simulink model "sgMdl_IO3xx_Serial_Loopback_Halfduplex"  (R2024b)
settings: Solver=FixedStepAuto  StartTime=0.0  StopTime=inf  RelTol=1e-3  EnableMultiTasking=on
undefined symbols (not defined in the file): Pull, pull, up
libraries: speedgoatlib_fpga_serial x6, simulink x2, speedgoatlib_interrupt x1, speedgoatlib_fpga x1
Description:
  | IO3xx Serial - Loopback Halfduplex
settings Model: ModifiedByFormat=Speedgoat  SimulationMode=external  ExtModeTrigDuration=100000  Creator=Speedgoat  LastModifiedBy=Speedgoat
settings SolverCC: ConcurrentTasks=on  AlgebraicLoopSolver=TrustRegion  PositivePriorityOrder=on  InsertRTBMode=Never (minimum delay)
settings DataIOCC: SaveFormat=Array  SaveState=on  SignalLoggingName=logsOut
settings OptimizationCC: BlockReduction=off  BooleanDataType=off  OptimizeBlockIOStorage=off  BufferReuse=off  ReuseModelBlockBuffer=off  GlobalBufferReuse=off  ExpressionFolding=off  LocalBlockOutputs=off  InitFltsAndDblsToZero=on  OptimizeDataStoreBuffers=off  BusAssignmentInplaceUpdate=off
settings DebuggingCC: SaveWithParameterizedLinksMsg=none  UnderspecifiedInitializationDetection=Classic  MergeDetectMultiDrivingBlocksExec=none  CheckExecutionContextPreStartOutputMsg=on  SignalResolutionControl=TryResolveAllWithWarning  TasksWithSamePriorityMsg=none  UnconnectedInputMsg=warning  UnconnectedOutputMsg=warning  UnconnectedLineMsg=warning  SFUnexpectedBacktrackingDiag=warning  SFNoUnconditionalDefaultTransitionDiag=warning  SFExecutionAtInitializationDiag=none  ArithmeticOperatorsInVariantConditions=warning
settings HardwareCC: ProdBitPerLong=64  ProdLongLongMode=on  ProdHWDeviceType=Intel->x86-64 (Linux 64)
settings ModelReferenceCC: EnableRefExpFcnMdlSchedulingChecks=on  PropagateSignalLabelsOutOfModel=off
settings SFSimCC: SimUseLocalCustomCode=off  SimTargetLang=C++
settings RTWCC: Description=Speedgoat Real-Time Target Machine  SystemTargetFile=speedgoat.tlc  TemplateMakefile=slrealtime_default_tmf  PostCodeGenCommand=sg.model.build.makeCfg(bdroot, buildInfo);  RTWUseLocalCustomCode=off  Toolchain=Simulink Real-Time Toolchain  BuildConfiguration=Faster Runs  TargetLang=C++  GPUComputeCapability=3.5  DLArmComputeVersion=19.05
settings CodeAppCC: StateflowObjectComments=on
settings SimulinkRealTimeTargetCC: SubcomponentCodeInterfacePackaging=Reusable function  MATLABClassNameForMDSCustomization=Simulink.SoftwareTarget.GRTCustomization  InstructionSetFMA=off  LogToMDFFile=off  SLRTFileLogMaxRuns=10  UseGCCFastMath=on
settings ConfigComp: CovMetricSettings=dw  CovSaveCumulativeToWorkspaceVar=on  CovSaveSingleToWorkspaceVar=on  CovExternalEMLEnable=off  CovSFcnEnable=off  CovBoundaryAbsTol=1.0e-5

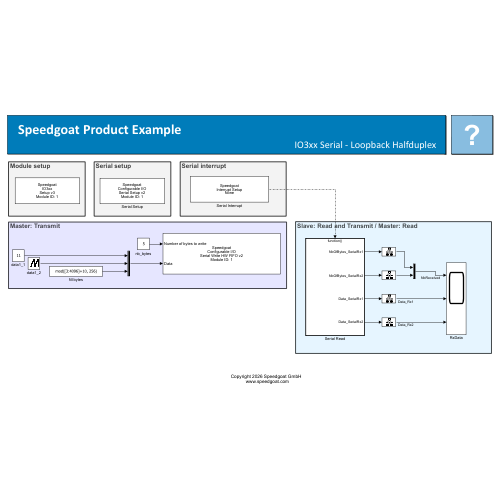
[thumbnail: Simulink's stored preview of the top-level diagram]
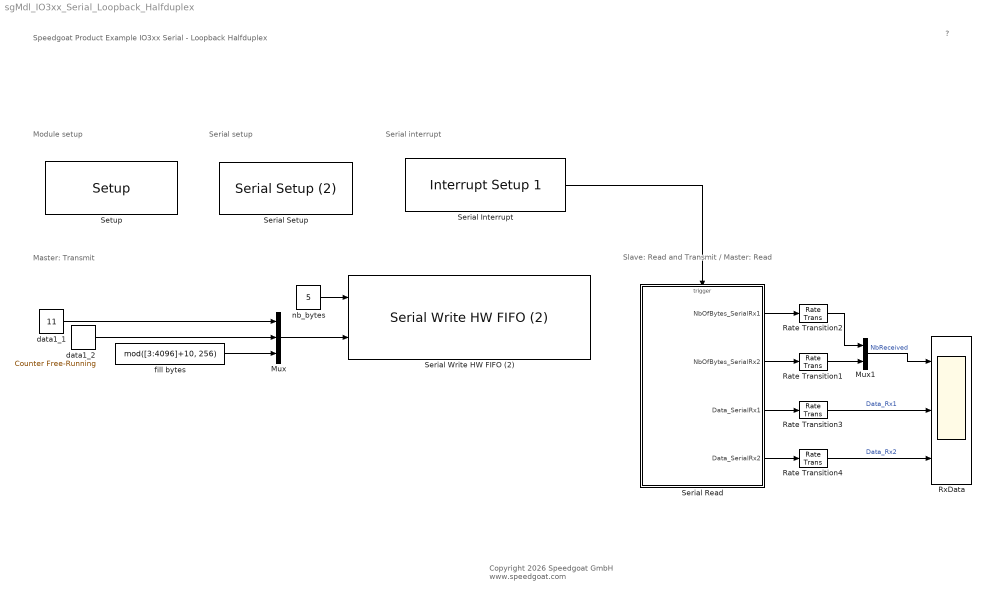
== system sgMdl_IO3xx_Serial_Loopback_Halfduplex ==
  note: Slave: Read and Transmit / Master: Read
  note: Master: Transmit
  note: Module setup
  note: Serial setup
  note: Serial interrupt
  note: Speedgoat Product Example
      | IO3xx Serial - Loopback Halfduplex
  note: ?
  note: Copyright 2026 Speedgoat GmbH
      |  www.speedgoat.com
  Mux : Mux  Inputs=3
  Mux1 : Mux  Inputs=2
  Rate Transition{1..4} (4 alike) : RateTransition  Deterministic=off
  RxData : Scope  NumInputPorts=3
  Serial Interrupt : speedgoatlib_interrupt/Interrupt Setup 1  parModuleTrigger=off  parPollingMode=off  parPriorityConf=High  parPriority=254  confStartFcn=IO324_200k_SERIAL_start_public  confStopFcn=IO324_200k_SERIAL_stop_public  confIsrFcn=IO324_200k_SERIAL_isr_public  confMapFcn=IO324_200k_SERIAL_map_public  confHookFile=io324_200k_serial_int_hooks.c  confIrqNr=-1  confIsPolling=off  confModID=16776961  confSelectedInt=None  confSelectedId=[]  confSelectedChannel=[]  confData=[]  confForcePollingMode=off
  Serial Read : Subsystem  TreatAsAtomicUnit=on
  Serial Setup : speedgoatlib_fpga_serial/Serial Setup (2)  id=1  channel=[1, 2]  bitrate=[1e6]  bitrate_effective=[996.3243e3, 996.3243e3]  bitrate_error=[-0.36757, -0.36757]  parity_mode=No parity  data_length=[8]  stop_length=[2]  enable_half_duplex=[0]  rx_character_timeout=[1 1]
      settings: SourceProductName=Simulink Real-Time: Speedgoat I/O Blockset
  Serial Write HW FIFO (2) : speedgoatlib_fpga_serial/Serial Write HW FIFO (2)  id=1  channel=1  ts=-1  data_length=8
      settings: SourceProductName=Simulink Real-Time: Speedgoat I/O Blockset
  Setup : speedgoatlib_fpga/Setup/Setup  board=Please select...  id=1  pciSlot=-1  device_id=1  bitstreamFilePath=C:\Work\SVN\Speedgoatlib\releases\10.0.0\product_examples\IO3xx_Serial  bitstreamFile=Please select...  fpgaFreq=[73728000 100000000]  enableDma=off  rearEnb_1=off  rearIO_1=None  rearEnb_2=off  rearIO_2=None  ProgSpiFlash=off  ProgBPIFlash=off  useFpgaDmaController=off  dmaTrigDropdown=Model Step  dmaTrigSelect=0  dmaStopOnOverload=on  dmaModeSequential=on  dmaModeParallel=off  PullRPort15=pull-up 3.3V  PullRPort31=pull-up 3.3V  PullRPort47=pull-up 3.3V  PullRPort63=pull-up 3.3V  diffLineTermination_1=on  diffLineTermination_2=on  diffLineTermination_3=on  diffLineTermination_4=on  diffLineTermination_5=on  diffLineTermination_6=on  diffLineTermination_7=on  diffLineTermination_8=on  diffLineTermination_9=on  diffLineTermination_10=on  diffLineTermination_11=on  diffLineTermination_12=on  diffLineTermination_13=on  diffLineTermination_14=on  diffLineTermination_15=on  diffLineTermination_16=on  diffLineTermination_17=on  diffLineTermination_18=on  diffLineTermination_19=on  diffLineTermination_20=on  diffLineTermination_21=on  diffLineTermination_22=on  diffLineTermination_23=on  diffLineTermination_24=on  diffLineTermination_25=on  diffLineTermination_26=on  diffLineTermination_27=on  diffLineTermination_28=on  diffLineTermination_29=on  diffLineTermination_30=on  diffLineTermination_31=on  diffLineTermination_32=on  ioVoltageDropDown1=3.3V  pullResistorDropDown1_1=Pull-up  pullResistorDropDown1_2=Pull-up  pullResistorDropDown1_3=Pull-up  pullResistorDropDown1_4=Pull-up  pullResistorDropDown1_5=Pull-up  pullResistorDropDown1_6=Pull-up  pullResistorDropDown1_7=Pull-up  pullResistorDropDown1_8=Pull-up  ttlIsImplementedCheckBox1=off  pullResistorDropDown2=Pull-up  ioVoltageDropDown2=3.3V  ttlIsImplementedCheckBox2=off  pullResistorDropDown3=Pull-up  ioVoltageDropDown3=3.3V  ttlIsImplementedCheckBox3=off  pullResistorDropDown4=Pull-up  ioVoltageDropDown4=3.3V  ttlIsImplementedCheckBox4=off  pullResistorDropDown5=Pull-up  ioVoltageDropDown5=3.3V  ttlIsImplementedCheckBox5=off  pullResistorDropDown6=Pull-up  ioVoltageDropDown6=3.3V  ttlIsImplementedCheckBox6=off  pullResistorDropDown7=Pull-up  ioVoltageDropDown7=3.3V  ttlIsImplementedCheckBox7=off  pullResistorDropDown8=Pull-up  ioVoltageDropDown8=3.3V  ttlIsImplementedCheckBox8=off  terminationCheckBox1=off  terminationCheckBox2=off  terminationCheckBox3=off  terminationCheckBox4=off  diffIsImplementedCheckBox1=off  terminationCheckBox5=off  terminationCheckBox6=off  terminationCheckBox7=off  terminationCheckBox8=off  diffIsImplementedCheckBox2=off  terminationCheckBox9=off  terminationCheckBox10=off  terminationCheckBox11=off  terminationCheckBox12=off  diffIsImplementedCheckBox3=off  terminationCheckBox13=off  terminationCheckBox14=off  terminationCheckBox15=off  terminationCheckBox16=off  diffIsImplementedCheckBox4=off  terminationCheckBox17=off  terminationCheckBox18=off  terminationCheckBox19=off  terminationCheckBox20=off  diffIsImplementedCheckBox5=off  terminationCheckBox21=off  terminationCheckBox22=off  terminationCheckBox23=off  terminationCheckBox24=off  diffIsImplementedCheckBox6=off  terminationCheckBox25=off  terminationCheckBox26=off  terminationCheckBox27=off  terminationCheckBox28=off  diffIsImplementedCheckBox7=off  terminationCheckBox29=off  terminationCheckBox30=off  terminationCheckBox31=off  terminationCheckBox32=off  diffIsImplementedCheckBox8=off  PullRPort0_1=pull-up  VioPort0_1=3.3V  PullRPort1_1=pull-up  VioPort1_1=3.3V  PullRPort2_1=pull-up  VioPort2_1=3.3V  PullRPort3_1=pull-up  VioPort3_1=3.3V  PullRPort4_1=pull-up  VioPort4_1=3.3V  PullRPort5_1=pull-up  VioPort5_1=3.3V  PullRPort6_1=pull-up  VioPort6_1=3.3V  diffLineTermination_rear1_1=on  diffLineTermination_rear1_2=on  diffLineTermination_rear1_3=on  diffLineTermination_rear1_4=on  diffLineTermination_rear1_5=on  diffLineTermination_rear1_6=on  diffLineTermination_rear1_7=on  diffLineTermination_rear1_8=on  PullRPort0_2=pull-up  VioPort0_2=3.3V  PullRPort1_2=pull-up  VioPort1_2=3.3V  PullRPort2_2=pull-up  VioPort2_2=3.3V  PullRPort3_2=pull-up  VioPort3_2=3.3V  PullRPort4_2=pull-up  VioPort4_2=3.3V  PullRPort5_2=pull-up  VioPort5_2=3.3V  PullRPort6_2=pull-up  VioPort6_2=3.3V  diffLineTermination_rear2_1=on  diffLineTermination_rear2_2=on  diffLineTermination_rear2_3=on  diffLineTermination_rear2_4=on  diffLineTermination_rear2_5=on  diffLineTermination_rear2_6=on  diffLineTermination_rear2_7=on  diffLineTermination_rear2_8=on
      settings: SourceProductName=Simulink Real-Time: Speedgoat I/O Blockset
  data1_1 : Constant  Value=11  OutDataTypeStr=Inherit: Inherit via back propagation
  data1_2 : simulink/Sources/Counter Free-Running  NumBits=8  tsamp=1e-3
  fill bytes : Constant  Value=mod([3:4096]+10, 256)  OutDataTypeStr=Inherit: Inherit via back propagation
  nb_bytes : Constant  Value=5  OutDataTypeStr=Inherit: Inherit via back propagation
      mask help: Speedgoat Utility Block<br>Interrupt Setup - Configure Speedgoat I/O Module interrupts<br><br>&copy; 2007 - 2026, Speedgoat GmbH, <a href="matlab: web('www.speedgoat.com','-browser');">www.speedgoat.com</a>
      mask Help: eval('sg.utils.help.show(''io_main/refentry_ref_interrupt_setup'');')
  wires:
  data1_1/1 -> Mux/1
  nb_bytes/1 -> Serial Write HW FIFO (2)/1
  Mux/1 -> Serial Write HW FIFO (2)/2
  Serial Read/4(Data_SerialRx2) -> Rate Transition4/1
  Serial Read/2(NbOfBytes_SerialRx2) -> Rate Transition1/1
  fill bytes/1 -> Mux/3
  Serial Read/1(NbOfBytes_SerialRx1) -> Rate Transition2/1
  Serial Read/3(Data_SerialRx1) -> Rate Transition3/1
  Serial Interrupt/1 -> Serial Read/Trigger
  data1_2/1 -> Mux/2
  Rate Transition4/1 -> RxData/3  "Data_Rx2"
  Rate Transition3/1 -> RxData/2  "Data_Rx1"
  Rate Transition1/1 -> Mux1/2
  Rate Transition2/1 -> Mux1/1
  Mux1/1 -> RxData/1  "NbReceived"

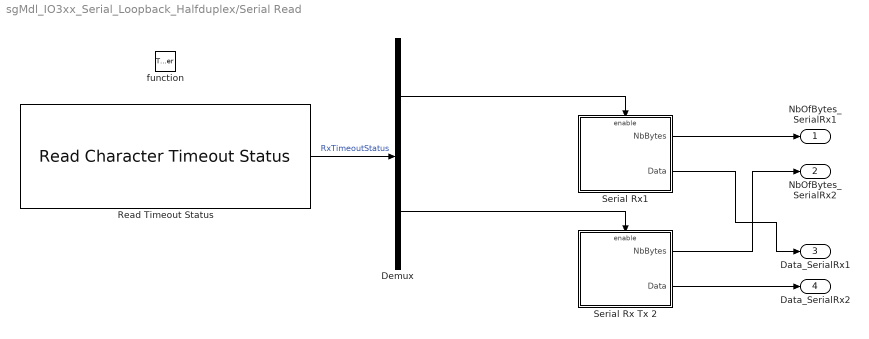
== system sgMdl_IO3xx_Serial_Loopback_Halfduplex/Serial Read ==
  function : TriggerPort  TriggerType=function-call  VariantControl=Variant
  Demux : Demux  Outputs=2
  Read Timeout Status : speedgoatlib_fpga_serial/Read Character Timeout Status  id=1  channel=[1, 2]  ts=-1
      settings: SourceProductName=Simulink Real-Time: Speedgoat I/O Blockset
  Serial Rx Tx 2 : Subsystem  TreatAsAtomicUnit=on
  Serial Rx1 : Subsystem  TreatAsAtomicUnit=on
  NbOfBytes_SerialRx1 : Outport
  NbOfBytes_SerialRx2 : Outport  Port=2
  Data_SerialRx1 : Outport  Port=3
  Data_SerialRx2 : Outport  Port=4
  wires:
  Serial Rx Tx 2/2(Data) -> Data_SerialRx2/1
  Serial Rx Tx 2/1(NbBytes) -> NbOfBytes_SerialRx2/1
  Demux/1 -> Serial Rx1/Enable
  Demux/2 -> Serial Rx Tx 2/Enable
  Read Timeout Status/1 -> Demux/1  "RxTimeoutStatus"
  Serial Rx1/1(NbBytes) -> NbOfBytes_SerialRx1/1
  Serial Rx1/2(Data) -> Data_SerialRx1/1

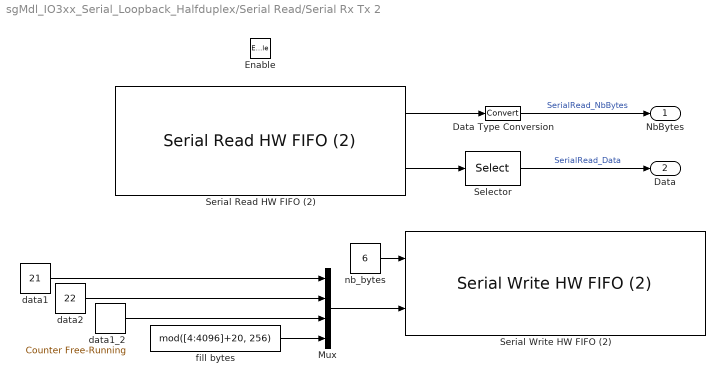
== system sgMdl_IO3xx_Serial_Loopback_Halfduplex/Serial Read/Serial Rx Tx 2 ==
  Enable : EnablePort
  Data Type Conversion : DataTypeConversion  SaturateOnIntegerOverflow=off  RndMeth=Floor
  Mux : Mux
  Selector : Selector  InputPortWidth=4096  IndexOptions=Index vector (dialog)  Indices=[1:5]  OutputSizes=1
  Serial Read HW FIFO (2) : speedgoatlib_fpga_serial/Serial Read HW FIFO (2)  id=1  channel=2  ts=-1  data_length=8
      settings: SourceProductName=Simulink Real-Time: Speedgoat I/O Blockset
  Serial Write HW FIFO (2) : speedgoatlib_fpga_serial/Serial Write HW FIFO (2)  id=1  channel=2  ts=-1  data_length=8
      settings: SourceProductName=Simulink Real-Time: Speedgoat I/O Blockset
  data1 : Constant  Value=21  OutDataTypeStr=Inherit: Inherit via back propagation  SampleTime=-1
  data1_2 : simulink/Sources/Counter Free-Running  NumBits=8  tsamp=-1
  data2 : Constant  Value=22  OutDataTypeStr=Inherit: Inherit via back propagation  SampleTime=-1
  fill bytes : Constant  Value=mod([4:4096]+20, 256)  OutDataTypeStr=Inherit: Inherit via back propagation  SampleTime=-1
  nb_bytes : Constant  Value=6  OutDataTypeStr=Inherit: Inherit via back propagation  SampleTime=-1
  NbBytes : Outport
  Data : Outport  Port=2
  wires:
  Serial Read HW FIFO (2)/2 -> Selector/1
  Selector/1 -> Data/1  "SerialRead_Data"
  Data Type Conversion/1 -> NbBytes/1  "SerialRead_NbBytes"
  Serial Read HW FIFO (2)/1 -> Data Type Conversion/1
  nb_bytes/1 -> Serial Write HW FIFO (2)/1
  data1_2/1 -> Mux/3
  fill bytes/1 -> Mux/4
  Mux/1 -> Serial Write HW FIFO (2)/2
  data1/1 -> Mux/1
  data2/1 -> Mux/2

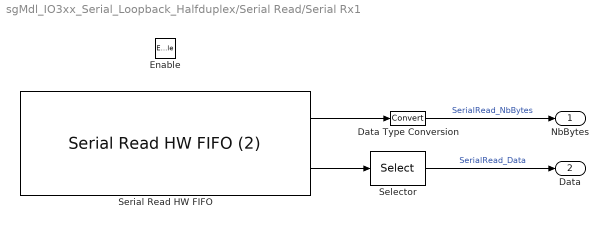
== system sgMdl_IO3xx_Serial_Loopback_Halfduplex/Serial Read/Serial Rx1 ==
  Enable : EnablePort
  Data Type Conversion : DataTypeConversion  SaturateOnIntegerOverflow=off  RndMeth=Floor
  Selector : Selector  InputPortWidth=4096  IndexOptions=Index vector (dialog)  Indices=[1:6]  OutputSizes=1
  Serial Read HW FIFO : speedgoatlib_fpga_serial/Serial Read HW FIFO (2)  id=1  channel=1  ts=-1  data_length=8
      settings: SourceProductName=Simulink Real-Time: Speedgoat I/O Blockset
  NbBytes : Outport
  Data : Outport  Port=2
  wires:
  Serial Read HW FIFO/1 -> Data Type Conversion/1
  Data Type Conversion/1 -> NbBytes/1  "SerialRead_NbBytes"
  Selector/1 -> Data/1  "SerialRead_Data"
  Serial Read HW FIFO/2 -> Selector/1
